simulink model "arduino_closed_loop_opcua"  (R2020b)
settings: Solver=VariableStepAuto  StartTime=0.0  StopTime=900  FixedStep=0.1  RelTol=1e-3
PreLoadFcn:
  | set_point=30;
  | kp=1.6;
  | ki=1/114.07;
libraries: pid_lib x1, realtime_pacer_lib x1
settings Model: Creator=Jonas  LastModifiedBy=churban
settings DataIOCC: ExternalInput=[uaClient]

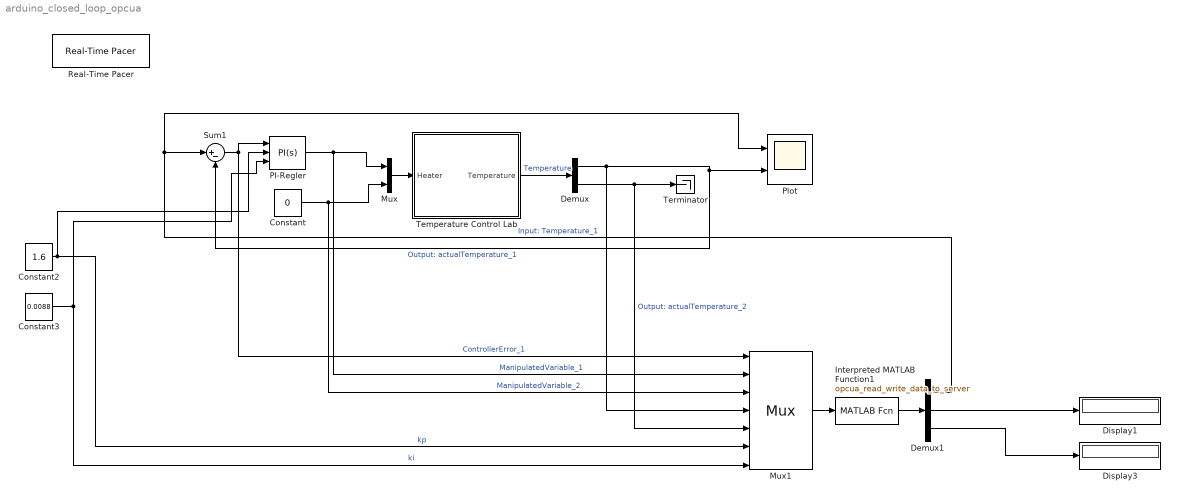
== system arduino_closed_loop_opcua ==
  Constant : Constant  Value=0
  Constant2 : Constant  Value=1.6
  Constant3 : Constant  Value=0.0088
  Demux : Demux  Outputs=2
  Demux1 : Demux  Outputs=3
  Display1 : Display
  Display3 : Display
  Interpreted MATLAB Function1 : MATLABFcn  MATLABFcn=opcua_read_write_data_to_server  OutputDimensions=3
  Mux : Mux  Inputs=2
  Mux1 : Mux  Inputs=7
      settings: DisplayOption=signals
  PI-Regler : pid_lib/PID Controller  Controller=PI  Form=Ideal  TimeDomain=Continuous-time  UseExternalTs=off  SampleTime=-1  IntegratorMethod=Forward Euler  FilterMethod=Forward Euler  ControllerParametersSource=external  P=1.6  I=0.0088  D=0  UseFilter=on  N=100  TunerSelectOption=Transfer Function Based (PID Tuner App)  ZeroCross=off  InitialConditionSource=internal  InitialConditionForIntegrator=0  InitialConditionForFilter=0  DifferentiatorICPrevScaledInput=0  ExternalReset=none  TrackingMode=off  Kt=1  LimitOutput=on  SatLimitsSource=internal  UpperSaturationLimit=80  LowerSaturationLimit=0  LinearizeAsGain=on  AntiWindupMode=none  Kb=1  POutMin=[]  POutMax=[]  IOutMin=[]  IOutMax=[]  DOutMin=[]  DOutMax=[]  NOutMin=[]  NOutMax=[]  SumOutMin=[]  SumOutMax=[]  SaturationOutMin=[]  SaturationOutMax=[]  PParamMin=[]  PParamMax=[]  IParamMin=[]  IParamMax=[]  DParamMin=[]  DParamMax=[]  NParamMin=[]  NParamMax=[]  KbParamMin=[]  KbParamMax=[]  KtParamMin=[]  KtParamMax=[]  KbOutMin=[]  KbOutMax=[]  KtOutMin=[]  KtOutMax=[]  IntegratorOutMin=[]  IntegratorOutMax=[]  FilterOutMin=[]  FilterOutMax=[]  SumI1OutMin=[]  SumI1OutMax=[]  SumI2OutMin=[]  SumI2OutMax=[]  SumI3OutMin=[]  SumI3OutMax=[]  SumI4OutMin=[]  SumI4OutMax=[]  SumDOutMin=[]  SumDOutMax=[]  DifferentiatorOutMin=[]  DifferentiatorOutMax=[]  FilterDiffOutCoefMin=[]  FilterDiffOutCoefMax=[]  ReciprocalOutMin=[]  ReciprocalOutMax=[]  SumDenOutMin=[]  SumDenOutMax=[]  SumNumOutMin=[]  SumNumOutMax=[]  DivideOutMin=[]  DivideOutMax=[]  UdiffTsProdOutMin=[]  UdiffTsProdOutMax=[]  NTsProdOutMin=[]  NTsProdOutMax=[]  UintegralTsProdOutMin=[]  UintegralTsProdOutMax=[]  UngainTsProdOutMin=[]  UngainTsProdOutMax=[]  IntegratorContinuousStateAttributes=''  IntegratorStateMustResolveToSignalObject=off  IntegratorRTWStateStorageClass=Auto  FilterContinuousStateAttributes=''  FilterStateMustResolveToSignalObject=off  FilterRTWStateStorageClass=Auto  ParallelPVariant=Passthrough  IdealPVariant=ExternalParameters  IVariant=ExternalParameters  DVariant=Disabled  IntegratorVariant=Continuous  SatVariant=Enabled  AWVariant=Passthrough  PCopyVariant=Disabled  TRVariant=Disabled  FdbkBlocksVariant=Forward  IdealPFdbkVariant=Disabled  SatFdbkVariant=Disabled  DerivativeFilterVariant=Disabled  NVariant=Disabled  NCopyVariant=Disabled_SignalSpec  FilterICVariant=Disabled  IntegratorICVariant=InternalICs  ExternalResetVariant=Disabled  TRSumVariant=Passthrough  SumFdbkVariant=Disabled  SumVariant=Sum_PI  TsampFilterVariant=InternalTs  TsampNgainVariant=Passthrough  TsampIntegralVariant=Passthrough  ExternalSaturationOutDataTypeStr=Inherit: Same as second input
  Plot : Scope  NumInputPorts=2
  Real-Time Pacer : realtime_pacer_lib/Real-Time Pacer  simTimePerRealTime=1
  Sum1 : Sum  Inputs=|+-
  Temperature Control Lab : Subsystem
  Terminator : Terminator
  wires:
  Sum1/1 -> PI-Regler/1, Mux1/1  "ControllerError_1"
  Demux1/1 -> Plot/1, Sum1/1  "Input: Temperature_1"
  PI-Regler/1 -> Mux1/2, Mux/1  "ManipulatedVariable_1"
  Demux/1 -> Mux1/4, Sum1/2, Plot/2  "Output: actualTemperature_1"
  Mux/1 -> Temperature Control Lab/1(Heater)
  Constant/1 -> Mux1/3, Mux/2  "ManipulatedVariable_2"
  Temperature Control Lab/1(Temperature) -> Demux/1  "Temperature"
  Demux/2 -> Mux1/5, Terminator/1  "Output: actualTemperature_2"
  Mux1/1 -> Interpreted MATLAB Function1/1
  Interpreted MATLAB Function1/1 -> Demux1/1
  Demux1/2 -> Display1/1
  Demux1/3 -> Display3/1
  Constant2/1 -> PI-Regler/2, Mux1/6  "kp"
  Constant3/1 -> PI-Regler/3, Mux1/7  "ki"

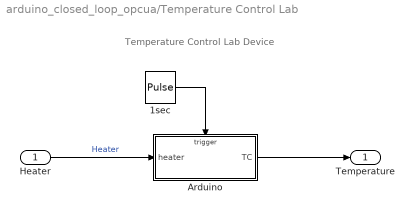
== system arduino_closed_loop_opcua/Temperature Control Lab ==
  note: Temperature Control Lab Device
  Heater : Inport
  1sec : DiscretePulseGenerator  PulseType=Time based  Period=1  PulseWidth=50
  Arduino : Subsystem  TreatAsAtomicUnit=on
  Temperature : Outport  VectorParamsAs1DForOutWhenUnconnected=off
  wires:
  1sec/1 -> Arduino/Trigger
  Arduino/1(TC) -> Temperature/1
  Heater/1 -> Arduino/1(heater)  "Heater"

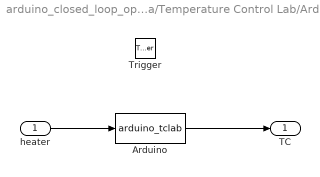
== system arduino_closed_loop_opcua/Temperature Control Lab/Arduino ==
  heater : Inport  LatchByDelayingOutsideSignal=on
  Trigger : TriggerPort  VariantControl=Variant
  Arduino : MATLABFcn  MATLABFcn=arduino_tclab
  TC : Outport  InitialOutput=[23 23]  VectorParamsAs1DForOutWhenUnconnected=off
  wires:
  heater/1 -> Arduino/1
  Arduino/1 -> TC/1
